simulink model "custom_model"  (R2017a)
settings: Solver=VariableStepAuto  StartTime=0.0  StopTime=10.0  RelTol=1e-3
settings Model: Creator=Vera  LastModifiedBy=Vera

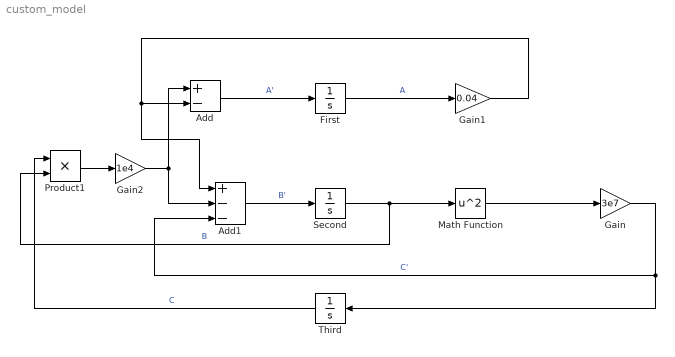
== system custom_model ==
  Add : Sum  Inputs=+-
  Add1 : Sum  Inputs=+--
  First : Integrator
  Gain : Gain  Gain=3e7
  Gain1 : Gain  Gain=0.04
  Gain2 : Gain  Gain=1e4
  Math Function : Math  Operator=square  SaturateOnIntegerOverflow=on
  Product1 : Product
  Second : Integrator
  Third : Integrator
  wires:
  Add/1 -> First/1  "A'"
  First/1 -> Gain1/1  "A"
  Add1/1 -> Second/1  "B'"
  Second/1 -> Product1/2, Math Function/1  "B"
  Math Function/1 -> Gain/1
  Gain1/1 -> Add1/1, Add/2
  Product1/1 -> Gain2/1
  Third/1 -> Product1/1  "C"
  Gain/1 -> Add1/3, Third/1  "C'"
  Gain2/1 -> Add/1, Add1/2
